simulink model "bus_as_currsource_charging_discharging_final_rearranged"  (R2023a)
settings: Solver=VariableStepAuto  StartTime=0.0  StopTime=10.0  RelTol=1e-3
libraries: spsParallelRLCBranchLib x72, spsCurrentMeasurementLib x27, spsVoltageMeasurementLib x27, spspowerguiLib x25, spsControlledVoltageSourceLib x24, spsVariableResistorLib x24, spsSeriesRLCBranchLib x6, spsMosfetLib x2, sdolib x1, spsControlledCurrentSourceLib x1, spsGroundLib x1
(part 1 of 4)
settings Model: Creator=Amith  LastModifiedBy=Amith

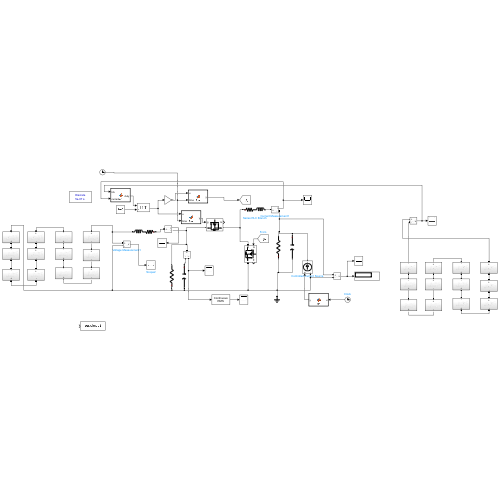
[thumbnail: Simulink's stored preview of the top-level diagram]
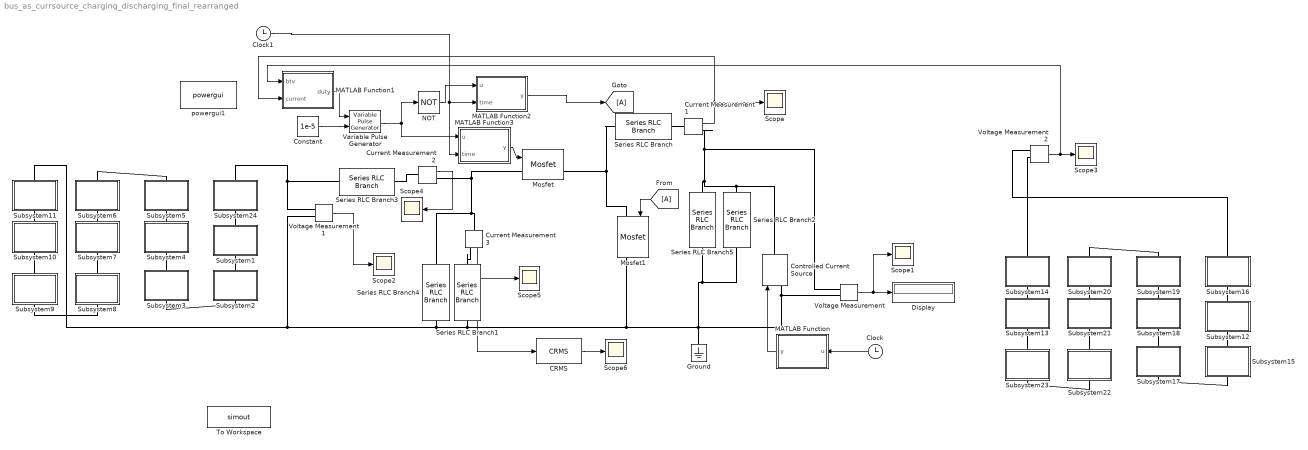
== system bus_as_currsource_charging_discharging_final_rearranged ==
  CRMS : sdolib/RMS Blocks/CRMS
  Clock : Clock
  Clock1 : Clock
  Constant : Constant  Value=1e-5
  Controlled Current Source : spsControlledCurrentSourceLib/Controlled Current Source  Initialize=on  Source_Type=AC  Amplitude=0  Phase=0  Frequency=0  Measurements=None
  Current Measurement1 : spsCurrentMeasurementLib/Current Measurement  PhasorSimulation=off  OutputType=Complex  PSBequivalent=0
  Current Measurement2 : spsCurrentMeasurementLib/Current Measurement  PhasorSimulation=off  OutputType=Complex  PSBequivalent=0
  Current Measurement3 : spsCurrentMeasurementLib/Current Measurement  PhasorSimulation=off  OutputType=Complex  PSBequivalent=0
  Display : Display
  From : From
  Goto : Goto
  Ground : spsGroundLib/Ground  LConnTagsString=a
  MATLAB Function : MATLAB Function  TreatAsAtomicUnit=on
  MATLAB Function1 : MATLAB Function  TreatAsAtomicUnit=on
  MATLAB Function2 : MATLAB Function  TreatAsAtomicUnit=on
  MATLAB Function3 : MATLAB Function  TreatAsAtomicUnit=on
  Mosfet : spsMosfetLib/Mosfet  Ron=0.1  Lon=0  Rd=0.01  Vfd=0  IC=0  Rs=1e5  Cs=inf  Measurements=on
  Mosfet1 : spsMosfetLib/Mosfet  Ron=0.1  Lon=0  Rd=0.01  Vfd=0  IC=0  Rs=1e5  Cs=inf  Measurements=on
  NOT : Logic  Operator=NOT  IconShape=distinctive  AllPortsSameDT=off  OutDataTypeStr=boolean
  Scope{,1..6} (7 alike) : Scope
  Series RLC Branch : spsSeriesRLCBranchLib/Series RLC Branch  LConnTagsString=__new0  RConnTagsString=__new0  BranchType=RL  Resistance=2.4e-3  Inductance=22e-6  SetiL0=off  InitialCurrent=0  Capacitance=1e-6  Setx0=off  InitialVoltage=0  Measurements=None
  Series RLC Branch1 : spsSeriesRLCBranchLib/Series RLC Branch  LConnTagsString=__new0  RConnTagsString=__new0  BranchType=C  Resistance=1  Inductance=1e-3  SetiL0=off  InitialCurrent=0  Capacitance=94e-6  Setx0=off  InitialVoltage=0  Measurements=None
  Series RLC Branch2 : spsSeriesRLCBranchLib/Series RLC Branch  LConnTagsString=__new0  RConnTagsString=__new0  BranchType=C  Resistance=1  Inductance=1e-3  SetiL0=off  InitialCurrent=0  Capacitance=188e-6  Setx0=off  InitialVoltage=0  Measurements=None
  Series RLC Branch3 : spsSeriesRLCBranchLib/Series RLC Branch  LConnTagsString=__new0  RConnTagsString=__new0  BranchType=RL  Resistance=2.4e-3  Inductance=22e-6  SetiL0=off  InitialCurrent=0  Capacitance=256.86e-6  Setx0=off  InitialVoltage=0  Measurements=None
  Series RLC Branch4 : spsSeriesRLCBranchLib/Series RLC Branch  LConnTagsString=__new0  RConnTagsString=__new0  BranchType=R  Resistance=10e3  Inductance=22e-6  SetiL0=off  InitialCurrent=0  Capacitance=256.86e-6  Setx0=off  InitialVoltage=0  Measurements=None
  Series RLC Branch5 : spsSeriesRLCBranchLib/Series RLC Branch  LConnTagsString=__new0  RConnTagsString=__new0  BranchType=R  Resistance=10e3  Inductance=22e-6  SetiL0=off  InitialCurrent=0  Capacitance=256.86e-6  Setx0=off  InitialVoltage=0  Measurements=None
  Subsystem1 : Subsystem
  Subsystem10 : Subsystem
  Subsystem11 : Subsystem
  Subsystem12 : Subsystem
  Subsystem13 : Subsystem
  Subsystem14 : Subsystem
  Subsystem15 : Subsystem
  Subsystem16 : Subsystem
  Subsystem17 : Subsystem
  Subsystem18 : Subsystem
  Subsystem19 : Subsystem
  Subsystem2 : Subsystem
  Subsystem20 : Subsystem
  Subsystem21 : Subsystem
  Subsystem22 : Subsystem
  Subsystem23 : Subsystem
  Subsystem24 : Subsystem
  Subsystem3 : Subsystem
  Subsystem4 : Subsystem
  Subsystem5 : Subsystem
  Subsystem6 : Subsystem
  Subsystem7 : Subsystem
  Subsystem8 : Subsystem
  Subsystem9 : Subsystem
  To Workspace : ToWorkspace  VariableName=simout  SaveFormat=Timeseries  SampleTime=-1
  Variable Pulse Generator : VariablePulseGenerator  SampleTime=0.1
  Voltage Measurement : spsVoltageMeasurementLib/Voltage Measurement  PhasorSimulation=off  OutputType=Complex  PSBequivalent=0
  Voltage Measurement1 : spsVoltageMeasurementLib/Voltage Measurement  PhasorSimulation=off  OutputType=Complex  PSBequivalent=0
  Voltage Measurement2 : spsVoltageMeasurementLib/Voltage Measurement  PhasorSimulation=off  OutputType=Complex  PSBequivalent=0
  powergui1 : spspowerguiLib/powergui  Priority=1  SimulationMode=Discrete  SampleTime=5e-7  frequency=60  Iterations=50  frequencyindice=0  Pbase=100e6  ErrMax=1e-4  UnitsV=kV  UnitsW=MW  buscounter=0  FunctionMessages=off  echomessages=off  EnableUseOfTLC=off  CurrentSourceSwitches=off  DisableSnubberDevices=off  DisableRonSwitches=off  DisableVfSwitches=off  DisplayEquations=off  AutomaticDiscreteSolvers=off  SolverType=Tustin/Backward Euler (TBE)  Interpol=off  ExternalGateDelay=off  methode=off  Ts=100  x0status=blocks  SPID=on  SwTol=0  HookPort=off  NonlinearTolerance=1e-4  nMaxIteration=100  ContinueOnMaxIteration=off  RestoreLinks=warning  ResistiveCurrentMeasurement=off  Frange=[0:2:500]  Ylog=off  Xlog=on  ShowGrid=off  save=off  variable=ZData  structure=0  ZoomFFT=off  StartTime=0.0  cycles=1  DisplayStyle=1  fundamental=60  FreqAxis=off  MaxFrequency=1000  frequencyindicesteady=1  RmsSteady=1  display=off
  wires:
  Voltage Measurement/1 -> Scope1/1, Display/1
  MATLAB Function1/1(duty) -> Variable Pulse Generator/1
  Clock/1 -> MATLAB Function/1(u)
  Current Measurement2/1 -> Scope4/1
  From/1 -> Mosfet1/1
  Constant/1 -> Variable Pulse Generator/2
  Current Measurement3/1 -> Scope5/1, CRMS/1
  CRMS/1 -> Scope6/1
  NOT/1 -> MATLAB Function2/1(u)
  Current Measurement1/1 -> Scope/1, MATLAB Function1/2(current)
  MATLAB Function2/1(y) -> Goto/1
  MATLAB Function/1(y) -> Controlled Current Source/1
  MATLAB Function3/1(y) -> Mosfet/1
  Clock1/1 -> MATLAB Function3/2(time), MATLAB Function2/2(time)
  Variable Pulse Generator/1 -> MATLAB Function3/1(u), NOT/1
  Voltage Measurement2/1 -> MATLAB Function1/1(btv), Scope3/1
  Voltage Measurement1/1 -> Scope2/1
  connections:
  Series RLC Branch2/RConn1 -- Voltage Measurement/LConn2 -- Controlled Current Source/LConn1 -- Ground/LConn1 -- Subsystem11/LConn1 -- Voltage Measurement1/LConn2 -- Series RLC Branch4/LConn1 -- Series RLC Branch1/RConn1 -- Mosfet1/RConn1 -- Series RLC Branch5/LConn1
  Current Measurement1/RConn1 -- Voltage Measurement/LConn1 -- Controlled Current Source/RConn1 -- Series RLC Branch2/LConn1 -- Series RLC Branch5/RConn1
  Series RLC Branch3/RConn1 -- Voltage Measurement1/LConn1 -- Subsystem24/RConn1
  Mosfet/RConn1 -- Mosfet1/LConn1 -- Series RLC Branch/LConn1
  Current Measurement3/LConn1 -- Series RLC Branch4/RConn1 -- Current Measurement2/RConn1 -- Mosfet/LConn1
  Subsystem15/LConn1 -- Subsystem17/RConn1
  Subsystem16/RConn1 -- Voltage Measurement2/LConn1
  Subsystem7/RConn1 -- Subsystem6/LConn1
  Subsystem8/LConn1 -- Subsystem9/RConn1
  Subsystem12/RConn1 -- Subsystem16/LConn1
  Subsystem22/LConn1 -- Subsystem23/RConn1
  Subsystem20/RConn1 -- Subsystem19/LConn1
  Subsystem8/RConn1 -- Subsystem7/LConn1
  Subsystem4/RConn1 -- Subsystem3/LConn1
  Subsystem2/RConn1 -- Subsystem1/LConn1
  Subsystem11/RConn1 -- Subsystem10/LConn1
  Subsystem13/RConn1 -- Subsystem23/LConn1
  Subsystem19/RConn1 -- Subsystem18/LConn1
  Subsystem14/RConn1 -- Subsystem13/LConn1
  Subsystem18/RConn1 -- Subsystem17/LConn1
  Current Measurement1/LConn1 -- Series RLC Branch/RConn1
  Subsystem5/RConn1 -- Subsystem4/LConn1
  Subsystem1/RConn1 -- Subsystem24/LConn1
  Subsystem10/RConn1 -- Subsystem9/LConn1
  Current Measurement2/LConn1 -- Series RLC Branch3/LConn1
  Subsystem15/RConn1 -- Subsystem12/LConn1
  Subsystem14/LConn1 -- Voltage Measurement2/LConn2
  Series RLC Branch1/LConn1 -- Current Measurement3/RConn1
  Subsystem22/RConn1 -- Subsystem21/LConn1
  Subsystem6/RConn1 -- Subsystem5/LConn1
  Subsystem3/RConn1 -- Subsystem2/LConn1
  Subsystem21/RConn1 -- Subsystem20/LConn1

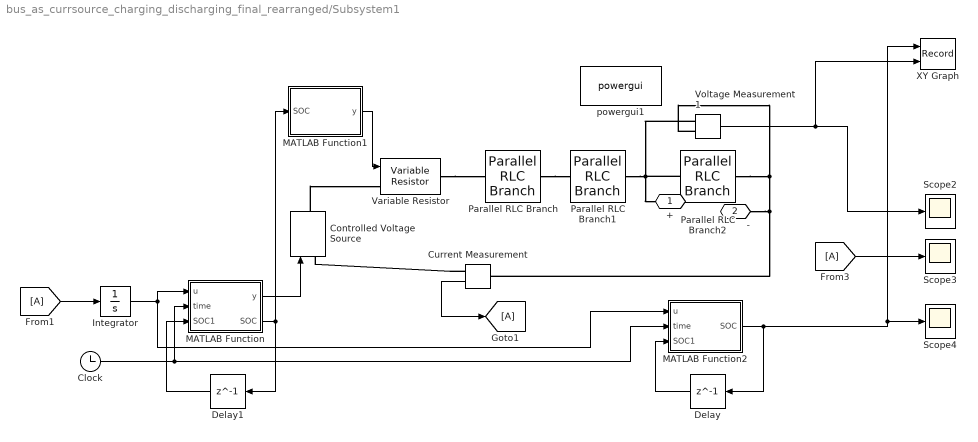
== system bus_as_currsource_charging_discharging_final_rearranged/Subsystem1 ==
  Clock : Clock
  Controlled Voltage Source : spsControlledVoltageSourceLib/Controlled Voltage Source  Initialize=on  Source_Type=DC  Amplitude=0  Phase=0  Frequency=0  Measurements=None
  Current Measurement : spsCurrentMeasurementLib/Current Measurement  PhasorSimulation=off  OutputType=Complex  PSBequivalent=0
  Delay : Delay  DelayLength=1  InitialCondition=0
  Delay1 : Delay  DelayLength=1  InitialCondition=0
  From1 : From
  From3 : From
  Goto1 : Goto
  Integrator : Integrator
  MATLAB Function : MATLAB Function  TreatAsAtomicUnit=on
  MATLAB Function1 : MATLAB Function  TreatAsAtomicUnit=on
  MATLAB Function2 : MATLAB Function  TreatAsAtomicUnit=on
  Parallel RLC Branch : spsParallelRLCBranchLib/Parallel RLC Branch  LConnTagsString=a  RConnTagsString=__new0  BranchType=RC  Resistance=15.5e-3  Inductance=1e-3  SetiL0=off  InitialCurrent=0  Capacitance=1028.7  Setx0=off  InitialVoltage=0  Measurements=None
  Parallel RLC Branch1 : spsParallelRLCBranchLib/Parallel RLC Branch  LConnTagsString=a  RConnTagsString=__new0  BranchType=RC  Resistance=18.3e-3  Inductance=1e-3  SetiL0=off  InitialCurrent=0  Capacitance=5756.6  Setx0=off  InitialVoltage=0  Measurements=None
  Parallel RLC Branch2 : spsParallelRLCBranchLib/Parallel RLC Branch  LConnTagsString=a  RConnTagsString=__new0  BranchType=R  Resistance=1e9  Inductance=1e-3  SetiL0=off  InitialCurrent=0  Capacitance=5756.6  Setx0=off  InitialVoltage=0  Measurements=None
  Scope2 : Scope
  Scope3 : Scope
  Scope4 : Scope
  Variable Resistor : spsVariableResistorLib/Variable Resistor  Rabsmin=1e-3
      settings: LibrarySourceBlock=sps_lib/Passives/Variable Resistor
  Voltage Measurement1 : spsVoltageMeasurementLib/Voltage Measurement  PhasorSimulation=off  OutputType=Complex  PSBequivalent=0
  XY Graph : Record  FileSettingsInternal="{\"entries\":[{\"content\":{\"excelSettings\":{\"content\":{},\"type\":\"Streamout.ExcelSettings\"}},\"type\":\"Streamout.FileSettingStorage\",\"uuid\":\"18842006-f205-45f0-aa2a-5042201a1171\"}],\"packageUris\":[\"http://schema.mathworks.com/mf0/streamout_blocks/R2020a\"],\"version\":\"1.0\"}"  Layout=[1 1]  SignalsInternal="{\"entries\":[{\"content\":{\"signals\":[{\"content\":{\"blockPath\":[\"untitled/Subsystem1/XY Graph\"],\"dimensions\":[1],\"domain\":\"untitled/Subsystem1/XY Graph\",\"lineColor\":\"#a2142f\",\"port\":1,\"signalID\":718,\"signalName\":\"MATLAB Function2\"},\"type\":\"RecordBlkView.Signal\",\"uuid\":\"8255158c-12c1-48e7-a974-9ade2a17e088\"},{\"content\":{\"blockPath\":[\"untitled/Subsystem1/XY Graph\"],\"dimensions\":[1],\"domain\":\"untitled/Subsystem1/XY Graph\",\"lineColor\":\"#139fff\",\"port\":2,\"signalID\":721,\"signalName\":\"Voltage Measurement1\"},\"type\":\"RecordBlkView.Signal\",\"uuid\":\"5dae4a47-f7fb-4179-ba61-09f1c7b2ee25\"}]},\"type\":\"RecordBlkView.InputSignals\",\"uuid\":\"df1e2d31-8fbb-4e56-9ead-2e4de2629ece\"}],\"packageUris\":[\"http://schema.mathworks.com/mf0/streamout_blocks/R2020a\"],\"version\":\"1.0\"}"  VisualizationBindings="{\"xyplotplugin\":{\"info\":[{\"series\":[],\"subplotID\":1}]}}"  CompatibilityTag=XY
  powergui1 : spspowerguiLib/powergui  Priority=1  SimulationMode=Discrete  SampleTime=2e-7  frequency=60  Iterations=50  frequencyindice=0  Pbase=100e6  ErrMax=1e-4  UnitsV=kV  UnitsW=MW  buscounter=0  FunctionMessages=off  echomessages=off  EnableUseOfTLC=off  CurrentSourceSwitches=off  DisableSnubberDevices=off  DisableRonSwitches=off  DisableVfSwitches=off  DisplayEquations=off  AutomaticDiscreteSolvers=off  SolverType=Tustin/Backward Euler (TBE)  Interpol=off  ExternalGateDelay=off  methode=off  Ts=100  x0status=blocks  SPID=on  SwTol=0  HookPort=off  NonlinearTolerance=1e-4  nMaxIteration=100  ContinueOnMaxIteration=off  RestoreLinks=warning  ResistiveCurrentMeasurement=off  Frange=[0:2:500]  Ylog=off  Xlog=on  ShowGrid=off  save=off  variable=ZData  structure=0  ZoomFFT=off  StartTime=0.0  cycles=1  DisplayStyle=1  fundamental=60  FreqAxis=off  MaxFrequency=1000  frequencyindicesteady=1  RmsSteady=1  display=off
  + : PMIOPort  Side=Right
  - : PMIOPort  Port=2  Side=Left
  wires:
  Current Measurement/1 -> Goto1/1
  From3/1 -> Scope3/1
  Voltage Measurement1/1 -> XY Graph/2, Scope2/1
  MATLAB Function2/1(SOC) -> Delay/1, XY Graph/1, Scope4/1
  From1/1 -> Integrator/1
  MATLAB Function/1(y) -> Controlled Voltage Source/1
  MATLAB Function1/1(y) -> Variable Resistor/1
  Integrator/1 -> MATLAB Function2/1(u), MATLAB Function/1(u)
  Clock/1 -> MATLAB Function2/2(time), MATLAB Function/2(time)
  MATLAB Function/2(SOC) -> Delay1/1, MATLAB Function1/1(SOC)
  Delay/1 -> MATLAB Function2/3(SOC1)
  Delay1/1 -> MATLAB Function/3(SOC1)
  connections:
  Variable Resistor/RConn1 -- Parallel RLC Branch/LConn1
  Parallel RLC Branch1/RConn1 -- Parallel RLC Branch2/LConn1 -- +/RConn1 -- Voltage Measurement1/LConn1
  Voltage Measurement1/LConn2 -- Parallel RLC Branch2/RConn1 -- -/RConn1 -- Current Measurement/LConn1
  Controlled Voltage Source/RConn1 -- Variable Resistor/LConn1
  Current Measurement/RConn1 -- Controlled Voltage Source/LConn1
  Parallel RLC Branch/RConn1 -- Parallel RLC Branch1/LConn1

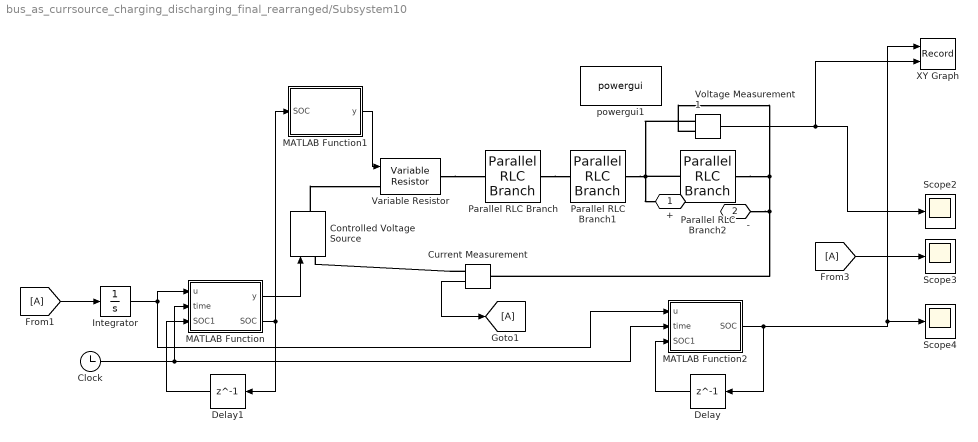
== system bus_as_currsource_charging_discharging_final_rearranged/Subsystem10 ==
  Clock : Clock
  Controlled Voltage Source : spsControlledVoltageSourceLib/Controlled Voltage Source  Initialize=on  Source_Type=DC  Amplitude=0  Phase=0  Frequency=0  Measurements=None
  Current Measurement : spsCurrentMeasurementLib/Current Measurement  PhasorSimulation=off  OutputType=Complex  PSBequivalent=0
  Delay : Delay  DelayLength=1  InitialCondition=0
  Delay1 : Delay  DelayLength=1  InitialCondition=0
  From1 : From
  From3 : From
  Goto1 : Goto
  Integrator : Integrator
  MATLAB Function : MATLAB Function  TreatAsAtomicUnit=on
  MATLAB Function1 : MATLAB Function  TreatAsAtomicUnit=on
  MATLAB Function2 : MATLAB Function  TreatAsAtomicUnit=on
  Parallel RLC Branch : spsParallelRLCBranchLib/Parallel RLC Branch  LConnTagsString=a  RConnTagsString=__new0  BranchType=RC  Resistance=15.5e-3  Inductance=1e-3  SetiL0=off  InitialCurrent=0  Capacitance=1028.7  Setx0=off  InitialVoltage=0  Measurements=None
  Parallel RLC Branch1 : spsParallelRLCBranchLib/Parallel RLC Branch  LConnTagsString=a  RConnTagsString=__new0  BranchType=RC  Resistance=18.3e-3  Inductance=1e-3  SetiL0=off  InitialCurrent=0  Capacitance=5756.6  Setx0=off  InitialVoltage=0  Measurements=None
  Parallel RLC Branch2 : spsParallelRLCBranchLib/Parallel RLC Branch  LConnTagsString=a  RConnTagsString=__new0  BranchType=R  Resistance=1e9  Inductance=1e-3  SetiL0=off  InitialCurrent=0  Capacitance=5756.6  Setx0=off  InitialVoltage=0  Measurements=None
  Scope2 : Scope
  Scope3 : Scope
  Scope4 : Scope
  Variable Resistor : spsVariableResistorLib/Variable Resistor  Rabsmin=1e-3
      settings: LibrarySourceBlock=sps_lib/Passives/Variable Resistor
  Voltage Measurement1 : spsVoltageMeasurementLib/Voltage Measurement  PhasorSimulation=off  OutputType=Complex  PSBequivalent=0
  XY Graph : Record  FileSettingsInternal="{\"entries\":[{\"content\":{\"excelSettings\":{\"content\":{},\"type\":\"Streamout.ExcelSettings\"}},\"type\":\"Streamout.FileSettingStorage\",\"uuid\":\"22b4d28b-aa9d-4c7b-bafe-c9a2b3ab8659\"}],\"packageUris\":[\"http://schema.mathworks.com/mf0/streamout_blocks/R2020a\"],\"version\":\"1.0\"}"  Layout=[1 1]  SignalsInternal="{\"entries\":[{\"content\":{\"signals\":[{\"content\":{\"blockPath\":[\"untitled/Subsystem10/XY Graph\"],\"dimensions\":[1],\"domain\":\"untitled/Subsystem10/XY Graph\",\"lineColor\":\"#ff6929\",\"port\":1,\"signalID\":726,\"signalName\":\"MATLAB Function2\"},\"type\":\"RecordBlkView.Signal\",\"uuid\":\"416f6dc6-347a-4c18-b72a-d27e661ecc55\"},{\"content\":{\"blockPath\":[\"untitled/Subsystem10/XY Graph\"],\"dimensions\":[1],\"domain\":\"untitled/Subsystem10/XY Graph\",\"lineColor\":\"#b746ff\",\"port\":2,\"signalID\":729,\"signalName\":\"Voltage Measurement1\"},\"type\":\"RecordBlkView.Signal\",\"uuid\":\"51357560-055d-4b10-b7e9-279a1a15faeb\"}]},\"type\":\"RecordBlkView.InputSignals\",\"uuid\":\"f10ebc27-9336-481b-9fb2-eb231a30c92e\"}],\"packageUris\":[\"http://schema.mathworks.com/mf0/streamout_blocks/R2020a\"],\"version\":\"1.0\"}"  VisualizationBindings="{\"xyplotplugin\":{\"info\":[{\"series\":[],\"subplotID\":1}]}}"  CompatibilityTag=XY
  powergui1 : spspowerguiLib/powergui  Priority=1  SimulationMode=Discrete  SampleTime=2e-7  frequency=60  Iterations=50  frequencyindice=0  Pbase=100e6  ErrMax=1e-4  UnitsV=kV  UnitsW=MW  buscounter=0  FunctionMessages=off  echomessages=off  EnableUseOfTLC=off  CurrentSourceSwitches=off  DisableSnubberDevices=off  DisableRonSwitches=off  DisableVfSwitches=off  DisplayEquations=off  AutomaticDiscreteSolvers=off  SolverType=Tustin/Backward Euler (TBE)  Interpol=off  ExternalGateDelay=off  methode=off  Ts=100  x0status=blocks  SPID=on  SwTol=0  HookPort=off  NonlinearTolerance=1e-4  nMaxIteration=100  ContinueOnMaxIteration=off  RestoreLinks=warning  ResistiveCurrentMeasurement=off  Frange=[0:2:500]  Ylog=off  Xlog=on  ShowGrid=off  save=off  variable=ZData  structure=0  ZoomFFT=off  StartTime=0.0  cycles=1  DisplayStyle=1  fundamental=60  FreqAxis=off  MaxFrequency=1000  frequencyindicesteady=1  RmsSteady=1  display=off
  + : PMIOPort  Side=Right
  - : PMIOPort  Port=2  Side=Left
  wires:
  Current Measurement/1 -> Goto1/1
  From3/1 -> Scope3/1
  Voltage Measurement1/1 -> XY Graph/2, Scope2/1
  MATLAB Function2/1(SOC) -> Delay/1, XY Graph/1, Scope4/1
  From1/1 -> Integrator/1
  MATLAB Function/1(y) -> Controlled Voltage Source/1
  MATLAB Function1/1(y) -> Variable Resistor/1
  Integrator/1 -> MATLAB Function2/1(u), MATLAB Function/1(u)
  Clock/1 -> MATLAB Function2/2(time), MATLAB Function/2(time)
  MATLAB Function/2(SOC) -> Delay1/1, MATLAB Function1/1(SOC)
  Delay/1 -> MATLAB Function2/3(SOC1)
  Delay1/1 -> MATLAB Function/3(SOC1)
  connections:
  Variable Resistor/RConn1 -- Parallel RLC Branch/LConn1
  Parallel RLC Branch1/RConn1 -- Parallel RLC Branch2/LConn1 -- +/RConn1 -- Voltage Measurement1/LConn1
  Voltage Measurement1/LConn2 -- Parallel RLC Branch2/RConn1 -- -/RConn1 -- Current Measurement/LConn1
  Controlled Voltage Source/RConn1 -- Variable Resistor/LConn1
  Current Measurement/RConn1 -- Controlled Voltage Source/LConn1
  Parallel RLC Branch/RConn1 -- Parallel RLC Branch1/LConn1

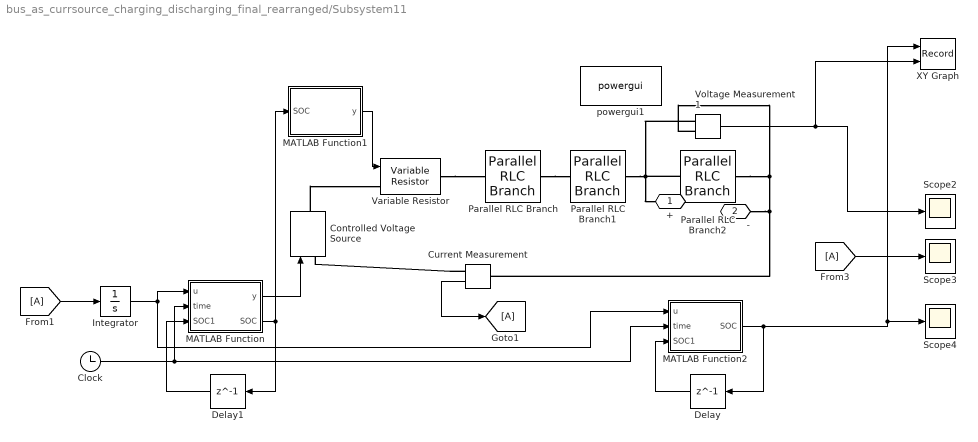
== system bus_as_currsource_charging_discharging_final_rearranged/Subsystem11 ==
  Clock : Clock
  Controlled Voltage Source : spsControlledVoltageSourceLib/Controlled Voltage Source  Initialize=on  Source_Type=DC  Amplitude=0  Phase=0  Frequency=0  Measurements=None
  Current Measurement : spsCurrentMeasurementLib/Current Measurement  PhasorSimulation=off  OutputType=Complex  PSBequivalent=0
  Delay : Delay  DelayLength=1  InitialCondition=0
  Delay1 : Delay  DelayLength=1  InitialCondition=0
  From1 : From
  From3 : From
  Goto1 : Goto
  Integrator : Integrator
  MATLAB Function : MATLAB Function  TreatAsAtomicUnit=on
  MATLAB Function1 : MATLAB Function  TreatAsAtomicUnit=on
  MATLAB Function2 : MATLAB Function  TreatAsAtomicUnit=on
  Parallel RLC Branch : spsParallelRLCBranchLib/Parallel RLC Branch  LConnTagsString=a  RConnTagsString=__new0  BranchType=RC  Resistance=15.5e-3  Inductance=1e-3  SetiL0=off  InitialCurrent=0  Capacitance=1028.7  Setx0=off  InitialVoltage=0  Measurements=None
  Parallel RLC Branch1 : spsParallelRLCBranchLib/Parallel RLC Branch  LConnTagsString=a  RConnTagsString=__new0  BranchType=RC  Resistance=18.3e-3  Inductance=1e-3  SetiL0=off  InitialCurrent=0  Capacitance=5756.6  Setx0=off  InitialVoltage=0  Measurements=None
  Parallel RLC Branch2 : spsParallelRLCBranchLib/Parallel RLC Branch  LConnTagsString=a  RConnTagsString=__new0  BranchType=R  Resistance=1e9  Inductance=1e-3  SetiL0=off  InitialCurrent=0  Capacitance=5756.6  Setx0=off  InitialVoltage=0  Measurements=None
  Scope2 : Scope
  Scope3 : Scope
  Scope4 : Scope
  Variable Resistor : spsVariableResistorLib/Variable Resistor  Rabsmin=1e-3
      settings: LibrarySourceBlock=sps_lib/Passives/Variable Resistor
  Voltage Measurement1 : spsVoltageMeasurementLib/Voltage Measurement  PhasorSimulation=off  OutputType=Complex  PSBequivalent=0
  XY Graph : Record  FileSettingsInternal="{\"entries\":[{\"content\":{\"excelSettings\":{\"content\":{},\"type\":\"Streamout.ExcelSettings\"}},\"type\":\"Streamout.FileSettingStorage\",\"uuid\":\"1c848b0b-adcf-4d1f-b91d-bbb3ed9b825d\"}],\"packageUris\":[\"http://schema.mathworks.com/mf0/streamout_blocks/R2020a\"],\"version\":\"1.0\"}"  Layout=[1 1]  SignalsInternal="{\"entries\":[{\"content\":{\"signals\":[{\"content\":{\"blockPath\":[\"untitled/Subsystem11/XY Graph\"],\"dimensions\":[1],\"domain\":\"untitled/Subsystem11/XY Graph\",\"lineColor\":\"#64d413\",\"port\":1,\"signalID\":734,\"signalName\":\"MATLAB Function2\"},\"type\":\"RecordBlkView.Signal\",\"uuid\":\"47c9a702-d54e-4048-aa36-620fba24fcff\"},{\"content\":{\"blockPath\":[\"untitled/Subsystem11/XY Graph\"],\"dimensions\":[1],\"domain\":\"untitled/Subsystem11/XY Graph\",\"lineColor\":\"#ff13a6\",\"port\":2,\"signalID\":737,\"signalName\":\"Voltage Measurement1\"},\"type\":\"RecordBlkView.Signal\",\"uuid\":\"f7e45941-7ce1-4a94-86f8-fd3d3864fbc4\"}]},\"type\":\"RecordBlkView.InputSignals\",\"uuid\":\"d32c99c7-d674-4a48-9e7c-b1b0ccc14c0d\"}],\"packageUris\":[\"http://schema.mathworks.com/mf0/streamout_blocks/R2020a\"],\"version\":\"1.0\"}"  VisualizationBindings="{\"xyplotplugin\":{\"info\":[{\"series\":[],\"subplotID\":1}]}}"  CompatibilityTag=XY
  powergui1 : spspowerguiLib/powergui  Priority=1  SimulationMode=Discrete  SampleTime=2e-7  frequency=60  Iterations=50  frequencyindice=0  Pbase=100e6  ErrMax=1e-4  UnitsV=kV  UnitsW=MW  buscounter=0  FunctionMessages=off  echomessages=off  EnableUseOfTLC=off  CurrentSourceSwitches=off  DisableSnubberDevices=off  DisableRonSwitches=off  DisableVfSwitches=off  DisplayEquations=off  AutomaticDiscreteSolvers=off  SolverType=Tustin/Backward Euler (TBE)  Interpol=off  ExternalGateDelay=off  methode=off  Ts=100  x0status=blocks  SPID=on  SwTol=0  HookPort=off  NonlinearTolerance=1e-4  nMaxIteration=100  ContinueOnMaxIteration=off  RestoreLinks=warning  ResistiveCurrentMeasurement=off  Frange=[0:2:500]  Ylog=off  Xlog=on  ShowGrid=off  save=off  variable=ZData  structure=0  ZoomFFT=off  StartTime=0.0  cycles=1  DisplayStyle=1  fundamental=60  FreqAxis=off  MaxFrequency=1000  frequencyindicesteady=1  RmsSteady=1  display=off
  + : PMIOPort  Side=Right
  - : PMIOPort  Port=2  Side=Left
  wires:
  Current Measurement/1 -> Goto1/1
  From3/1 -> Scope3/1
  Voltage Measurement1/1 -> XY Graph/2, Scope2/1
  MATLAB Function2/1(SOC) -> Delay/1, XY Graph/1, Scope4/1
  From1/1 -> Integrator/1
  MATLAB Function/1(y) -> Controlled Voltage Source/1
  MATLAB Function1/1(y) -> Variable Resistor/1
  Integrator/1 -> MATLAB Function2/1(u), MATLAB Function/1(u)
  Clock/1 -> MATLAB Function2/2(time), MATLAB Function/2(time)
  MATLAB Function/2(SOC) -> Delay1/1, MATLAB Function1/1(SOC)
  Delay/1 -> MATLAB Function2/3(SOC1)
  Delay1/1 -> MATLAB Function/3(SOC1)
  connections:
  Variable Resistor/RConn1 -- Parallel RLC Branch/LConn1
  Parallel RLC Branch1/RConn1 -- Parallel RLC Branch2/LConn1 -- +/RConn1 -- Voltage Measurement1/LConn1
  Voltage Measurement1/LConn2 -- Parallel RLC Branch2/RConn1 -- -/RConn1 -- Current Measurement/LConn1
  Controlled Voltage Source/RConn1 -- Variable Resistor/LConn1
  Current Measurement/RConn1 -- Controlled Voltage Source/LConn1
  Parallel RLC Branch/RConn1 -- Parallel RLC Branch1/LConn1

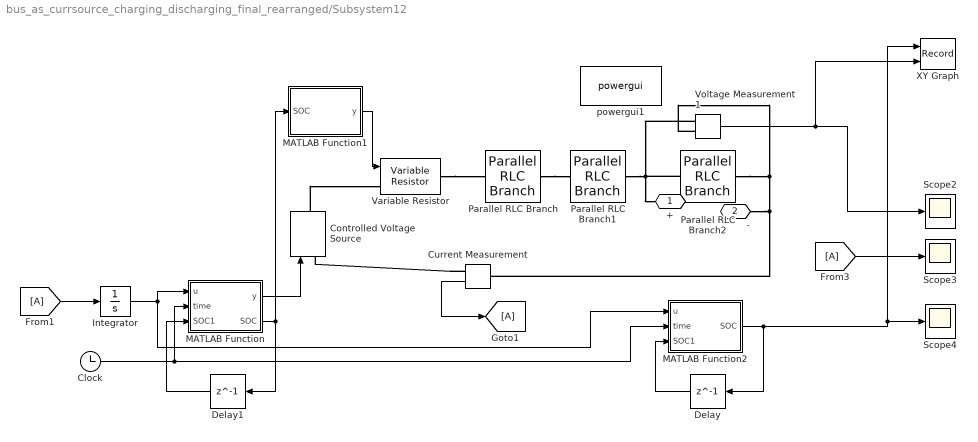
== system bus_as_currsource_charging_discharging_final_rearranged/Subsystem12 ==
  Clock : Clock
  Controlled Voltage Source : spsControlledVoltageSourceLib/Controlled Voltage Source  Initialize=on  Source_Type=DC  Amplitude=0  Phase=0  Frequency=0  Measurements=None
  Current Measurement : spsCurrentMeasurementLib/Current Measurement  PhasorSimulation=off  OutputType=Complex  PSBequivalent=0
  Delay : Delay  DelayLength=1  InitialCondition=0
  Delay1 : Delay  DelayLength=1  InitialCondition=0
  From1 : From
  From3 : From
  Goto1 : Goto
  Integrator : Integrator
  MATLAB Function : MATLAB Function  TreatAsAtomicUnit=on
  MATLAB Function1 : MATLAB Function  TreatAsAtomicUnit=on
  MATLAB Function2 : MATLAB Function  TreatAsAtomicUnit=on
  Parallel RLC Branch : spsParallelRLCBranchLib/Parallel RLC Branch  LConnTagsString=a  RConnTagsString=__new0  BranchType=RC  Resistance=15.5e-3  Inductance=1e-3  SetiL0=off  InitialCurrent=0  Capacitance=1028.7  Setx0=off  InitialVoltage=0  Measurements=None
  Parallel RLC Branch1 : spsParallelRLCBranchLib/Parallel RLC Branch  LConnTagsString=a  RConnTagsString=__new0  BranchType=RC  Resistance=18.3e-3  Inductance=1e-3  SetiL0=off  InitialCurrent=0  Capacitance=5756.6  Setx0=off  InitialVoltage=0  Measurements=None
  Parallel RLC Branch2 : spsParallelRLCBranchLib/Parallel RLC Branch  LConnTagsString=a  RConnTagsString=__new0  BranchType=R  Resistance=1e9  Inductance=1e-3  SetiL0=off  InitialCurrent=0  Capacitance=5756.6  Setx0=off  InitialVoltage=0  Measurements=None
  Scope2 : Scope
  Scope3 : Scope
  Scope4 : Scope
  Variable Resistor : spsVariableResistorLib/Variable Resistor  Rabsmin=1e-3
      settings: LibrarySourceBlock=sps_lib/Passives/Variable Resistor
  Voltage Measurement1 : spsVoltageMeasurementLib/Voltage Measurement  PhasorSimulation=off  OutputType=Complex  PSBequivalent=0
  XY Graph : Record  FileSettingsInternal="{\"entries\":[{\"content\":{\"excelSettings\":{\"content\":{},\"type\":\"Streamout.ExcelSettings\"}},\"type\":\"Streamout.FileSettingStorage\",\"uuid\":\"0f2e6bc2-adc7-4f2f-b180-28a43c082b9a\"}],\"packageUris\":[\"http://schema.mathworks.com/mf0/streamout_blocks/R2020a\"],\"version\":\"1.0\"}"  Layout=[1 1]  SignalsInternal="{\"entries\":[{\"content\":{\"signals\":[{\"content\":{\"blockPath\":[\"untitled/Subsystem12/XY Graph\"],\"dimensions\":[1],\"domain\":\"untitled/Subsystem12/XY Graph\",\"lineColor\":\"#fe330a\",\"port\":1,\"signalID\":742,\"signalName\":\"MATLAB Function2\"},\"type\":\"RecordBlkView.Signal\",\"uuid\":\"ea5ffbeb-f673-49b5-8228-f57bc36c2a28\"},{\"content\":{\"blockPath\":[\"untitled/Subsystem12/XY Graph\"],\"dimensions\":[1],\"domain\":\"untitled/Subsystem12/XY Graph\",\"lineColor\":\"#22b573\",\"port\":2,\"signalID\":745,\"signalName\":\"Voltage Measurement1\"},\"type\":\"RecordBlkView.Signal\",\"uuid\":\"e027727c-edef-4d69-b6da-103e96f1fdd0\"}]},\"type\":\"RecordBlkView.InputSignals\",\"uuid\":\"816a9515-beeb-4015-a901-a01888038e5f\"}],\"packageUris\":[\"http://schema.mathworks.com/mf0/streamout_blocks/R2020a\"],\"version\":\"1.0\"}"  VisualizationBindings="{\"xyplotplugin\":{\"info\":[{\"series\":[],\"subplotID\":1}]}}"  CompatibilityTag=XY
  powergui1 : spspowerguiLib/powergui  Priority=1  SimulationMode=Discrete  SampleTime=2e-7  frequency=60  Iterations=50  frequencyindice=0  Pbase=100e6  ErrMax=1e-4  UnitsV=kV  UnitsW=MW  buscounter=0  FunctionMessages=off  echomessages=off  EnableUseOfTLC=off  CurrentSourceSwitches=off  DisableSnubberDevices=off  DisableRonSwitches=off  DisableVfSwitches=off  DisplayEquations=off  AutomaticDiscreteSolvers=off  SolverType=Tustin/Backward Euler (TBE)  Interpol=off  ExternalGateDelay=off  methode=off  Ts=100  x0status=blocks  SPID=on  SwTol=0  HookPort=off  NonlinearTolerance=1e-4  nMaxIteration=100  ContinueOnMaxIteration=off  RestoreLinks=warning  ResistiveCurrentMeasurement=off  Frange=[0:2:500]  Ylog=off  Xlog=on  ShowGrid=off  save=off  variable=ZData  structure=0  ZoomFFT=off  StartTime=0.0  cycles=1  DisplayStyle=1  fundamental=60  FreqAxis=off  MaxFrequency=1000  frequencyindicesteady=1  RmsSteady=1  display=off
  + : PMIOPort  Side=Right
  - : PMIOPort  Port=2  Side=Left
  wires:
  Current Measurement/1 -> Goto1/1
  From3/1 -> Scope3/1
  Voltage Measurement1/1 -> XY Graph/2, Scope2/1
  MATLAB Function2/1(SOC) -> Delay/1, XY Graph/1, Scope4/1
  From1/1 -> Integrator/1
  MATLAB Function/1(y) -> Controlled Voltage Source/1
  MATLAB Function1/1(y) -> Variable Resistor/1
  Integrator/1 -> MATLAB Function2/1(u), MATLAB Function/1(u)
  Clock/1 -> MATLAB Function2/2(time), MATLAB Function/2(time)
  MATLAB Function/2(SOC) -> Delay1/1, MATLAB Function1/1(SOC)
  Delay/1 -> MATLAB Function2/3(SOC1)
  Delay1/1 -> MATLAB Function/3(SOC1)
  connections:
  Variable Resistor/RConn1 -- Parallel RLC Branch/LConn1
  Parallel RLC Branch1/RConn1 -- Parallel RLC Branch2/LConn1 -- +/RConn1 -- Voltage Measurement1/LConn1
  Voltage Measurement1/LConn2 -- Parallel RLC Branch2/RConn1 -- -/RConn1 -- Current Measurement/LConn1
  Controlled Voltage Source/RConn1 -- Variable Resistor/LConn1
  Current Measurement/RConn1 -- Controlled Voltage Source/LConn1
  Parallel RLC Branch/RConn1 -- Parallel RLC Branch1/LConn1

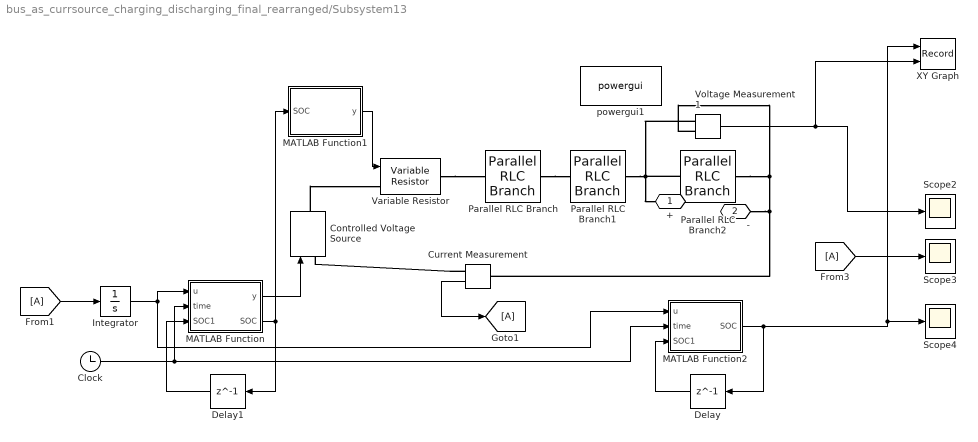
== system bus_as_currsource_charging_discharging_final_rearranged/Subsystem13 ==
  Clock : Clock
  Controlled Voltage Source : spsControlledVoltageSourceLib/Controlled Voltage Source  Initialize=on  Source_Type=DC  Amplitude=0  Phase=0  Frequency=0  Measurements=None
  Current Measurement : spsCurrentMeasurementLib/Current Measurement  PhasorSimulation=off  OutputType=Complex  PSBequivalent=0
  Delay : Delay  DelayLength=1  InitialCondition=0
  Delay1 : Delay  DelayLength=1  InitialCondition=0
  From1 : From
  From3 : From
  Goto1 : Goto
  Integrator : Integrator
  MATLAB Function : MATLAB Function  TreatAsAtomicUnit=on
  MATLAB Function1 : MATLAB Function  TreatAsAtomicUnit=on
  MATLAB Function2 : MATLAB Function  TreatAsAtomicUnit=on
  Parallel RLC Branch : spsParallelRLCBranchLib/Parallel RLC Branch  LConnTagsString=a  RConnTagsString=__new0  BranchType=RC  Resistance=15.5e-3  Inductance=1e-3  SetiL0=off  InitialCurrent=0  Capacitance=1028.7  Setx0=off  InitialVoltage=0  Measurements=None
  Parallel RLC Branch1 : spsParallelRLCBranchLib/Parallel RLC Branch  LConnTagsString=a  RConnTagsString=__new0  BranchType=RC  Resistance=18.3e-3  Inductance=1e-3  SetiL0=off  InitialCurrent=0  Capacitance=5756.6  Setx0=off  InitialVoltage=0  Measurements=None
  Parallel RLC Branch2 : spsParallelRLCBranchLib/Parallel RLC Branch  LConnTagsString=a  RConnTagsString=__new0  BranchType=R  Resistance=1e9  Inductance=1e-3  SetiL0=off  InitialCurrent=0  Capacitance=5756.6  Setx0=off  InitialVoltage=0  Measurements=None
  Scope2 : Scope
  Scope3 : Scope
  Scope4 : Scope
  Variable Resistor : spsVariableResistorLib/Variable Resistor  Rabsmin=1e-3
      settings: LibrarySourceBlock=sps_lib/Passives/Variable Resistor
  Voltage Measurement1 : spsVoltageMeasurementLib/Voltage Measurement  PhasorSimulation=off  OutputType=Complex  PSBequivalent=0
  XY Graph : Record  FileSettingsInternal="{\"entries\":[{\"content\":{\"excelSettings\":{\"content\":{},\"type\":\"Streamout.ExcelSettings\"}},\"type\":\"Streamout.FileSettingStorage\",\"uuid\":\"46f2ea04-5cee-4a3f-bbd1-60b3e0321189\"}],\"packageUris\":[\"http://schema.mathworks.com/mf0/streamout_blocks/R2020a\"],\"version\":\"1.0\"}"  Layout=[1 1]  SignalsInternal="{\"entries\":[{\"content\":{\"signals\":[{\"content\":{\"blockPath\":[\"untitled/Subsystem13/XY Graph\"],\"dimensions\":[1],\"domain\":\"untitled/Subsystem13/XY Graph\",\"lineColor\":\"#0072bd\",\"port\":1,\"signalID\":750,\"signalName\":\"MATLAB Function2\"},\"type\":\"RecordBlkView.Signal\",\"uuid\":\"17a12a08-f5f2-4398-835d-df73d8301e60\"},{\"content\":{\"blockPath\":[\"untitled/Subsystem13/XY Graph\"],\"dimensions\":[1],\"domain\":\"untitled/Subsystem13/XY Graph\",\"lineColor\":\"#d95319\",\"port\":2,\"signalID\":753,\"signalName\":\"Voltage Measurement1\"},\"type\":\"RecordBlkView.Signal\",\"uuid\":\"64892386-6769-470e-a7d8-214f68453155\"}]},\"type\":\"RecordBlkView.InputSignals\",\"uuid\":\"950e3db8-19c7-46df-8e03-320c742ac139\"}],\"packageUris\":[\"http://schema.mathworks.com/mf0/streamout_blocks/R2020a\"],\"version\":\"1.0\"}"  VisualizationBindings="{\"xyplotplugin\":{\"info\":[{\"series\":[],\"subplotID\":1}]}}"  CompatibilityTag=XY
  powergui1 : spspowerguiLib/powergui  Priority=1  SimulationMode=Discrete  SampleTime=2e-7  frequency=60  Iterations=50  frequencyindice=0  Pbase=100e6  ErrMax=1e-4  UnitsV=kV  UnitsW=MW  buscounter=0  FunctionMessages=off  echomessages=off  EnableUseOfTLC=off  CurrentSourceSwitches=off  DisableSnubberDevices=off  DisableRonSwitches=off  DisableVfSwitches=off  DisplayEquations=off  AutomaticDiscreteSolvers=off  SolverType=Tustin/Backward Euler (TBE)  Interpol=off  ExternalGateDelay=off  methode=off  Ts=100  x0status=blocks  SPID=on  SwTol=0  HookPort=off  NonlinearTolerance=1e-4  nMaxIteration=100  ContinueOnMaxIteration=off  RestoreLinks=warning  ResistiveCurrentMeasurement=off  Frange=[0:2:500]  Ylog=off  Xlog=on  ShowGrid=off  save=off  variable=ZData  structure=0  ZoomFFT=off  StartTime=0.0  cycles=1  DisplayStyle=1  fundamental=60  FreqAxis=off  MaxFrequency=1000  frequencyindicesteady=1  RmsSteady=1  display=off
  + : PMIOPort  Side=Right
  - : PMIOPort  Port=2  Side=Left
  wires:
  Current Measurement/1 -> Goto1/1
  From3/1 -> Scope3/1
  Voltage Measurement1/1 -> XY Graph/2, Scope2/1
  MATLAB Function2/1(SOC) -> Delay/1, XY Graph/1, Scope4/1
  From1/1 -> Integrator/1
  MATLAB Function/1(y) -> Controlled Voltage Source/1
  MATLAB Function1/1(y) -> Variable Resistor/1
  Integrator/1 -> MATLAB Function2/1(u), MATLAB Function/1(u)
  Clock/1 -> MATLAB Function2/2(time), MATLAB Function/2(time)
  MATLAB Function/2(SOC) -> Delay1/1, MATLAB Function1/1(SOC)
  Delay/1 -> MATLAB Function2/3(SOC1)
  Delay1/1 -> MATLAB Function/3(SOC1)
  connections:
  Variable Resistor/RConn1 -- Parallel RLC Branch/LConn1
  Parallel RLC Branch1/RConn1 -- Parallel RLC Branch2/LConn1 -- +/RConn1 -- Voltage Measurement1/LConn1
  Voltage Measurement1/LConn2 -- Parallel RLC Branch2/RConn1 -- -/RConn1 -- Current Measurement/LConn1
  Controlled Voltage Source/RConn1 -- Variable Resistor/LConn1
  Current Measurement/RConn1 -- Controlled Voltage Source/LConn1
  Parallel RLC Branch/RConn1 -- Parallel RLC Branch1/LConn1

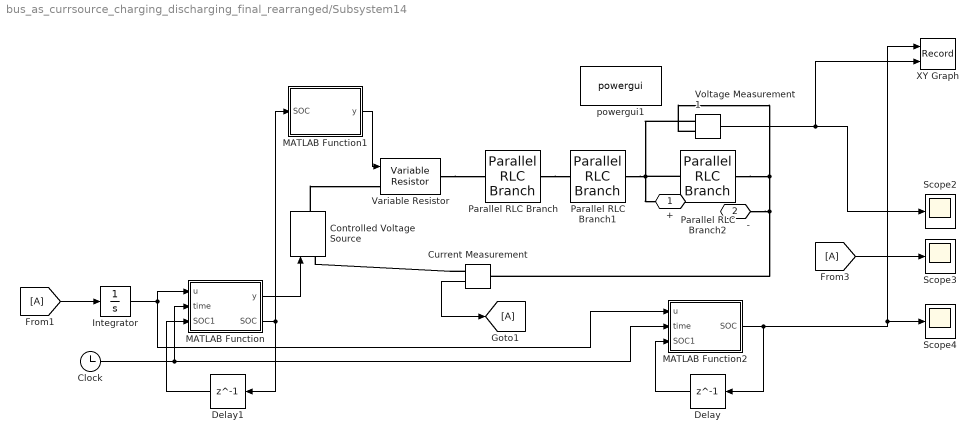
== system bus_as_currsource_charging_discharging_final_rearranged/Subsystem14 ==
  Clock : Clock
  Controlled Voltage Source : spsControlledVoltageSourceLib/Controlled Voltage Source  Initialize=on  Source_Type=DC  Amplitude=0  Phase=0  Frequency=0  Measurements=None
  Current Measurement : spsCurrentMeasurementLib/Current Measurement  PhasorSimulation=off  OutputType=Complex  PSBequivalent=0
  Delay : Delay  DelayLength=1  InitialCondition=0
  Delay1 : Delay  DelayLength=1  InitialCondition=0
  From1 : From
  From3 : From
  Goto1 : Goto
  Integrator : Integrator
  MATLAB Function : MATLAB Function  TreatAsAtomicUnit=on
  MATLAB Function1 : MATLAB Function  TreatAsAtomicUnit=on
  MATLAB Function2 : MATLAB Function  TreatAsAtomicUnit=on
  Parallel RLC Branch : spsParallelRLCBranchLib/Parallel RLC Branch  LConnTagsString=a  RConnTagsString=__new0  BranchType=RC  Resistance=15.5e-3  Inductance=1e-3  SetiL0=off  InitialCurrent=0  Capacitance=1028.7  Setx0=off  InitialVoltage=0  Measurements=None
  Parallel RLC Branch1 : spsParallelRLCBranchLib/Parallel RLC Branch  LConnTagsString=a  RConnTagsString=__new0  BranchType=RC  Resistance=18.3e-3  Inductance=1e-3  SetiL0=off  InitialCurrent=0  Capacitance=5756.6  Setx0=off  InitialVoltage=0  Measurements=None
  Parallel RLC Branch2 : spsParallelRLCBranchLib/Parallel RLC Branch  LConnTagsString=a  RConnTagsString=__new0  BranchType=R  Resistance=1e9  Inductance=1e-3  SetiL0=off  InitialCurrent=0  Capacitance=5756.6  Setx0=off  InitialVoltage=0  Measurements=None
  Scope2 : Scope
  Scope3 : Scope
  Scope4 : Scope
  Variable Resistor : spsVariableResistorLib/Variable Resistor  Rabsmin=1e-3
      settings: LibrarySourceBlock=sps_lib/Passives/Variable Resistor
  Voltage Measurement1 : spsVoltageMeasurementLib/Voltage Measurement  PhasorSimulation=off  OutputType=Complex  PSBequivalent=0
  XY Graph : Record  FileSettingsInternal="{\"entries\":[{\"content\":{\"excelSettings\":{\"content\":{},\"type\":\"Streamout.ExcelSettings\"}},\"type\":\"Streamout.FileSettingStorage\",\"uuid\":\"33cd7e7e-cb3e-43fd-8af6-a1cd50dbb10c\"}],\"packageUris\":[\"http://schema.mathworks.com/mf0/streamout_blocks/R2020a\"],\"version\":\"1.0\"}"  Layout=[1 1]  SignalsInternal="{\"entries\":[{\"content\":{\"signals\":[{\"content\":{\"blockPath\":[\"untitled/Subsystem14/XY Graph\"],\"dimensions\":[1],\"domain\":\"untitled/Subsystem14/XY Graph\",\"lineColor\":\"#edb120\",\"port\":1,\"signalID\":758,\"signalName\":\"MATLAB Function2\"},\"type\":\"RecordBlkView.Signal\",\"uuid\":\"8d895311-2c35-4cbd-8deb-b3bbf5e6af65\"},{\"content\":{\"blockPath\":[\"untitled/Subsystem14/XY Graph\"],\"dimensions\":[1],\"domain\":\"untitled/Subsystem14/XY Graph\",\"lineColor\":\"#7e2f8e\",\"port\":2,\"signalID\":761,\"signalName\":\"Voltage Measurement1\"},\"type\":\"RecordBlkView.Signal\",\"uuid\":\"c8704904-ac01-4b23-b785-d814eb32b585\"}]},\"type\":\"RecordBlkView.InputSignals\",\"uuid\":\"24ffd32b-dee3-4fd5-8e55-47aa3769188f\"}],\"packageUris\":[\"http://schema.mathworks.com/mf0/streamout_blocks/R2020a\"],\"version\":\"1.0\"}"  VisualizationBindings="{\"xyplotplugin\":{\"info\":[{\"series\":[],\"subplotID\":1}]}}"  CompatibilityTag=XY
  powergui1 : spspowerguiLib/powergui  Priority=1  SimulationMode=Discrete  SampleTime=2e-7  frequency=60  Iterations=50  frequencyindice=0  Pbase=100e6  ErrMax=1e-4  UnitsV=kV  UnitsW=MW  buscounter=0  FunctionMessages=off  echomessages=off  EnableUseOfTLC=off  CurrentSourceSwitches=off  DisableSnubberDevices=off  DisableRonSwitches=off  DisableVfSwitches=off  DisplayEquations=off  AutomaticDiscreteSolvers=off  SolverType=Tustin/Backward Euler (TBE)  Interpol=off  ExternalGateDelay=off  methode=off  Ts=100  x0status=blocks  SPID=on  SwTol=0  HookPort=off  NonlinearTolerance=1e-4  nMaxIteration=100  ContinueOnMaxIteration=off  RestoreLinks=warning  ResistiveCurrentMeasurement=off  Frange=[0:2:500]  Ylog=off  Xlog=on  ShowGrid=off  save=off  variable=ZData  structure=0  ZoomFFT=off  StartTime=0.0  cycles=1  DisplayStyle=1  fundamental=60  FreqAxis=off  MaxFrequency=1000  frequencyindicesteady=1  RmsSteady=1  display=off
  + : PMIOPort  Side=Right
  - : PMIOPort  Port=2  Side=Left
  wires:
  Current Measurement/1 -> Goto1/1
  From3/1 -> Scope3/1
  Voltage Measurement1/1 -> XY Graph/2, Scope2/1
  MATLAB Function2/1(SOC) -> Delay/1, XY Graph/1, Scope4/1
  From1/1 -> Integrator/1
  MATLAB Function/1(y) -> Controlled Voltage Source/1
  MATLAB Function1/1(y) -> Variable Resistor/1
  Integrator/1 -> MATLAB Function2/1(u), MATLAB Function/1(u)
  Clock/1 -> MATLAB Function2/2(time), MATLAB Function/2(time)
  MATLAB Function/2(SOC) -> Delay1/1, MATLAB Function1/1(SOC)
  Delay/1 -> MATLAB Function2/3(SOC1)
  Delay1/1 -> MATLAB Function/3(SOC1)
  connections:
  Variable Resistor/RConn1 -- Parallel RLC Branch/LConn1
  Parallel RLC Branch1/RConn1 -- Parallel RLC Branch2/LConn1 -- +/RConn1 -- Voltage Measurement1/LConn1
  Voltage Measurement1/LConn2 -- Parallel RLC Branch2/RConn1 -- -/RConn1 -- Current Measurement/LConn1
  Controlled Voltage Source/RConn1 -- Variable Resistor/LConn1
  Current Measurement/RConn1 -- Controlled Voltage Source/LConn1
  Parallel RLC Branch/RConn1 -- Parallel RLC Branch1/LConn1

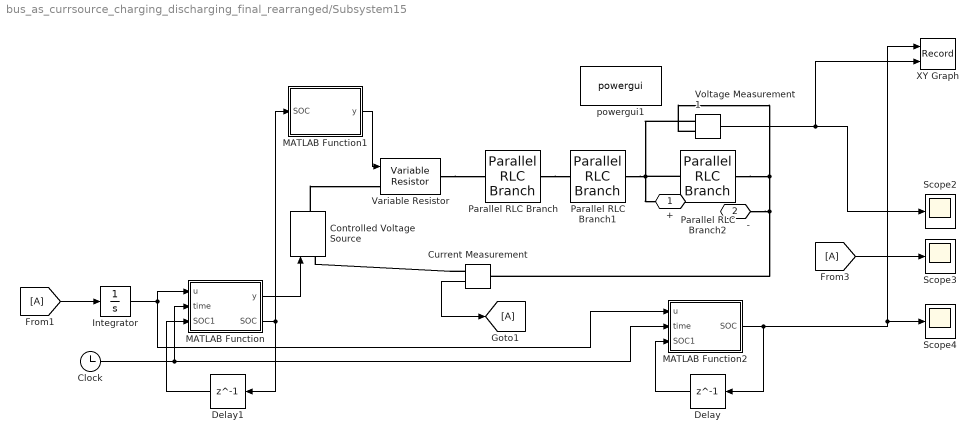
== system bus_as_currsource_charging_discharging_final_rearranged/Subsystem15 ==
  Clock : Clock
  Controlled Voltage Source : spsControlledVoltageSourceLib/Controlled Voltage Source  Initialize=on  Source_Type=DC  Amplitude=0  Phase=0  Frequency=0  Measurements=None
  Current Measurement : spsCurrentMeasurementLib/Current Measurement  PhasorSimulation=off  OutputType=Complex  PSBequivalent=0
  Delay : Delay  DelayLength=1  InitialCondition=0
  Delay1 : Delay  DelayLength=1  InitialCondition=0
  From1 : From
  From3 : From
  Goto1 : Goto
  Integrator : Integrator
  MATLAB Function : MATLAB Function  TreatAsAtomicUnit=on
  MATLAB Function1 : MATLAB Function  TreatAsAtomicUnit=on
  MATLAB Function2 : MATLAB Function  TreatAsAtomicUnit=on
  Parallel RLC Branch : spsParallelRLCBranchLib/Parallel RLC Branch  LConnTagsString=a  RConnTagsString=__new0  BranchType=RC  Resistance=15.5e-3  Inductance=1e-3  SetiL0=off  InitialCurrent=0  Capacitance=1028.7  Setx0=off  InitialVoltage=0  Measurements=None
  Parallel RLC Branch1 : spsParallelRLCBranchLib/Parallel RLC Branch  LConnTagsString=a  RConnTagsString=__new0  BranchType=RC  Resistance=18.3e-3  Inductance=1e-3  SetiL0=off  InitialCurrent=0  Capacitance=5756.6  Setx0=off  InitialVoltage=0  Measurements=None
  Parallel RLC Branch2 : spsParallelRLCBranchLib/Parallel RLC Branch  LConnTagsString=a  RConnTagsString=__new0  BranchType=R  Resistance=1e9  Inductance=1e-3  SetiL0=off  InitialCurrent=0  Capacitance=5756.6  Setx0=off  InitialVoltage=0  Measurements=None
  Scope2 : Scope
  Scope3 : Scope
  Scope4 : Scope
  Variable Resistor : spsVariableResistorLib/Variable Resistor  Rabsmin=1e-3
      settings: LibrarySourceBlock=sps_lib/Passives/Variable Resistor
  Voltage Measurement1 : spsVoltageMeasurementLib/Voltage Measurement  PhasorSimulation=off  OutputType=Complex  PSBequivalent=0
  XY Graph : Record  FileSettingsInternal="{\"entries\":[{\"content\":{\"excelSettings\":{\"content\":{},\"type\":\"Streamout.ExcelSettings\"}},\"type\":\"Streamout.FileSettingStorage\",\"uuid\":\"403cc223-e81b-4aa3-ab44-486a1f29fc47\"}],\"packageUris\":[\"http://schema.mathworks.com/mf0/streamout_blocks/R2020a\"],\"version\":\"1.0\"}"  Layout=[1 1]  SignalsInternal="{\"entries\":[{\"content\":{\"signals\":[{\"content\":{\"blockPath\":[\"untitled/Subsystem15/XY Graph\"],\"dimensions\":[1],\"domain\":\"untitled/Subsystem15/XY Graph\",\"lineColor\":\"#77ac30\",\"port\":1,\"signalID\":766,\"signalName\":\"MATLAB Function2\"},\"type\":\"RecordBlkView.Signal\",\"uuid\":\"c1a02276-32d7-41d4-a72a-c0476e60f96a\"},{\"content\":{\"blockPath\":[\"untitled/Subsystem15/XY Graph\"],\"dimensions\":[1],\"domain\":\"untitled/Subsystem15/XY Graph\",\"lineColor\":\"#4dbeee\",\"port\":2,\"signalID\":769,\"signalName\":\"Voltage Measurement1\"},\"type\":\"RecordBlkView.Signal\",\"uuid\":\"275a4661-1bcd-43c3-94eb-8eab3d22e323\"}]},\"type\":\"RecordBlkView.InputSignals\",\"uuid\":\"257ef280-70f4-4a70-9552-3d2113a1f719\"}],\"packageUris\":[\"http://schema.mathworks.com/mf0/streamout_blocks/R2020a\"],\"version\":\"1.0\"}"  VisualizationBindings="{\"xyplotplugin\":{\"info\":[{\"series\":[],\"subplotID\":1}]}}"  CompatibilityTag=XY
  powergui1 : spspowerguiLib/powergui  Priority=1  SimulationMode=Discrete  SampleTime=2e-7  frequency=60  Iterations=50  frequencyindice=0  Pbase=100e6  ErrMax=1e-4  UnitsV=kV  UnitsW=MW  buscounter=0  FunctionMessages=off  echomessages=off  EnableUseOfTLC=off  CurrentSourceSwitches=off  DisableSnubberDevices=off  DisableRonSwitches=off  DisableVfSwitches=off  DisplayEquations=off  AutomaticDiscreteSolvers=off  SolverType=Tustin/Backward Euler (TBE)  Interpol=off  ExternalGateDelay=off  methode=off  Ts=100  x0status=blocks  SPID=on  SwTol=0  HookPort=off  NonlinearTolerance=1e-4  nMaxIteration=100  ContinueOnMaxIteration=off  RestoreLinks=warning  ResistiveCurrentMeasurement=off  Frange=[0:2:500]  Ylog=off  Xlog=on  ShowGrid=off  save=off  variable=ZData  structure=0  ZoomFFT=off  StartTime=0.0  cycles=1  DisplayStyle=1  fundamental=60  FreqAxis=off  MaxFrequency=1000  frequencyindicesteady=1  RmsSteady=1  display=off
  + : PMIOPort  Side=Right
  - : PMIOPort  Port=2  Side=Left
  wires:
  Current Measurement/1 -> Goto1/1
  From3/1 -> Scope3/1
  Voltage Measurement1/1 -> XY Graph/2, Scope2/1
  MATLAB Function2/1(SOC) -> Delay/1, XY Graph/1, Scope4/1
  From1/1 -> Integrator/1
  MATLAB Function/1(y) -> Controlled Voltage Source/1
  MATLAB Function1/1(y) -> Variable Resistor/1
  Integrator/1 -> MATLAB Function2/1(u), MATLAB Function/1(u)
  Clock/1 -> MATLAB Function2/2(time), MATLAB Function/2(time)
  MATLAB Function/2(SOC) -> Delay1/1, MATLAB Function1/1(SOC)
  Delay/1 -> MATLAB Function2/3(SOC1)
  Delay1/1 -> MATLAB Function/3(SOC1)
  connections:
  Variable Resistor/RConn1 -- Parallel RLC Branch/LConn1
  Parallel RLC Branch1/RConn1 -- Parallel RLC Branch2/LConn1 -- +/RConn1 -- Voltage Measurement1/LConn1
  Voltage Measurement1/LConn2 -- Parallel RLC Branch2/RConn1 -- -/RConn1 -- Current Measurement/LConn1
  Controlled Voltage Source/RConn1 -- Variable Resistor/LConn1
  Current Measurement/RConn1 -- Controlled Voltage Source/LConn1
  Parallel RLC Branch/RConn1 -- Parallel RLC Branch1/LConn1

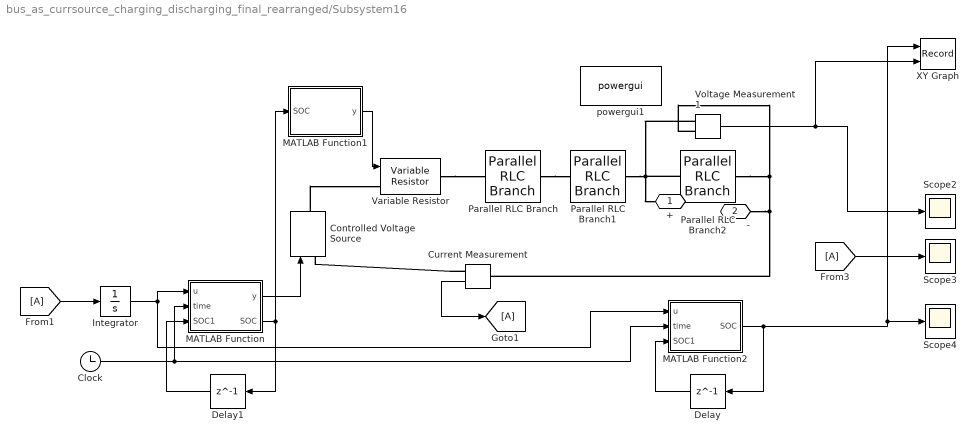
== system bus_as_currsource_charging_discharging_final_rearranged/Subsystem16 ==
  Clock : Clock
  Controlled Voltage Source : spsControlledVoltageSourceLib/Controlled Voltage Source  Initialize=on  Source_Type=DC  Amplitude=0  Phase=0  Frequency=0  Measurements=None
  Current Measurement : spsCurrentMeasurementLib/Current Measurement  PhasorSimulation=off  OutputType=Complex  PSBequivalent=0
  Delay : Delay  DelayLength=1  InitialCondition=0
  Delay1 : Delay  DelayLength=1  InitialCondition=0
  From1 : From
  From3 : From
  Goto1 : Goto
  Integrator : Integrator
  MATLAB Function : MATLAB Function  TreatAsAtomicUnit=on
  MATLAB Function1 : MATLAB Function  TreatAsAtomicUnit=on
  MATLAB Function2 : MATLAB Function  TreatAsAtomicUnit=on
  Parallel RLC Branch : spsParallelRLCBranchLib/Parallel RLC Branch  LConnTagsString=a  RConnTagsString=__new0  BranchType=RC  Resistance=15.5e-3  Inductance=1e-3  SetiL0=off  InitialCurrent=0  Capacitance=1028.7  Setx0=off  InitialVoltage=0  Measurements=None
  Parallel RLC Branch1 : spsParallelRLCBranchLib/Parallel RLC Branch  LConnTagsString=a  RConnTagsString=__new0  BranchType=RC  Resistance=18.3e-3  Inductance=1e-3  SetiL0=off  InitialCurrent=0  Capacitance=5756.6  Setx0=off  InitialVoltage=0  Measurements=None
  Parallel RLC Branch2 : spsParallelRLCBranchLib/Parallel RLC Branch  LConnTagsString=a  RConnTagsString=__new0  BranchType=R  Resistance=1e9  Inductance=1e-3  SetiL0=off  InitialCurrent=0  Capacitance=5756.6  Setx0=off  InitialVoltage=0  Measurements=None
  Scope2 : Scope
  Scope3 : Scope
  Scope4 : Scope
  Variable Resistor : spsVariableResistorLib/Variable Resistor  Rabsmin=1e-3
      settings: LibrarySourceBlock=sps_lib/Passives/Variable Resistor
  Voltage Measurement1 : spsVoltageMeasurementLib/Voltage Measurement  PhasorSimulation=off  OutputType=Complex  PSBequivalent=0
  XY Graph : Record  FileSettingsInternal="{\"entries\":[{\"content\":{\"excelSettings\":{\"content\":{},\"type\":\"Streamout.ExcelSettings\"}},\"type\":\"Streamout.FileSettingStorage\",\"uuid\":\"635a8de4-9d68-4305-8374-c64c95cd4a88\"}],\"packageUris\":[\"http://schema.mathworks.com/mf0/streamout_blocks/R2020a\"],\"version\":\"1.0\"}"  Layout=[1 1]  SignalsInternal="{\"entries\":[{\"content\":{\"signals\":[{\"content\":{\"blockPath\":[\"untitled/Subsystem16/XY Graph\"],\"dimensions\":[1],\"domain\":\"untitled/Subsystem16/XY Graph\",\"lineColor\":\"#a2142f\",\"port\":1,\"signalID\":774,\"signalName\":\"MATLAB Function2\"},\"type\":\"RecordBlkView.Signal\",\"uuid\":\"4a7bc012-1bee-4532-adb5-a858f4fb98a9\"},{\"content\":{\"blockPath\":[\"untitled/Subsystem16/XY Graph\"],\"dimensions\":[1],\"domain\":\"untitled/Subsystem16/XY Graph\",\"lineColor\":\"#139fff\",\"port\":2,\"signalID\":777,\"signalName\":\"Voltage Measurement1\"},\"type\":\"RecordBlkView.Signal\",\"uuid\":\"7f67f342-12e1-4167-85bc-002c2461bfa9\"}]},\"type\":\"RecordBlkView.InputSignals\",\"uuid\":\"2abac92f-8a54-481c-8c63-d11d4257a30b\"}],\"packageUris\":[\"http://schema.mathworks.com/mf0/streamout_blocks/R2020a\"],\"version\":\"1.0\"}"  VisualizationBindings="{\"xyplotplugin\":{\"info\":[{\"series\":[],\"subplotID\":1}]}}"  CompatibilityTag=XY
  powergui1 : spspowerguiLib/powergui  Priority=1  SimulationMode=Discrete  SampleTime=2e-7  frequency=60  Iterations=50  frequencyindice=0  Pbase=100e6  ErrMax=1e-4  UnitsV=kV  UnitsW=MW  buscounter=0  FunctionMessages=off  echomessages=off  EnableUseOfTLC=off  CurrentSourceSwitches=off  DisableSnubberDevices=off  DisableRonSwitches=off  DisableVfSwitches=off  DisplayEquations=off  AutomaticDiscreteSolvers=off  SolverType=Tustin/Backward Euler (TBE)  Interpol=off  ExternalGateDelay=off  methode=off  Ts=100  x0status=blocks  SPID=on  SwTol=0  HookPort=off  NonlinearTolerance=1e-4  nMaxIteration=100  ContinueOnMaxIteration=off  RestoreLinks=warning  ResistiveCurrentMeasurement=off  Frange=[0:2:500]  Ylog=off  Xlog=on  ShowGrid=off  save=off  variable=ZData  structure=0  ZoomFFT=off  StartTime=0.0  cycles=1  DisplayStyle=1  fundamental=60  FreqAxis=off  MaxFrequency=1000  frequencyindicesteady=1  RmsSteady=1  display=off
  + : PMIOPort  Side=Right
  - : PMIOPort  Port=2  Side=Left
  wires:
  Current Measurement/1 -> Goto1/1
  From3/1 -> Scope3/1
  Voltage Measurement1/1 -> XY Graph/2, Scope2/1
  MATLAB Function2/1(SOC) -> Delay/1, XY Graph/1, Scope4/1
  From1/1 -> Integrator/1
  MATLAB Function/1(y) -> Controlled Voltage Source/1
  MATLAB Function1/1(y) -> Variable Resistor/1
  Integrator/1 -> MATLAB Function2/1(u), MATLAB Function/1(u)
  Clock/1 -> MATLAB Function2/2(time), MATLAB Function/2(time)
  MATLAB Function/2(SOC) -> Delay1/1, MATLAB Function1/1(SOC)
  Delay/1 -> MATLAB Function2/3(SOC1)
  Delay1/1 -> MATLAB Function/3(SOC1)
  connections:
  Variable Resistor/RConn1 -- Parallel RLC Branch/LConn1
  Parallel RLC Branch1/RConn1 -- Parallel RLC Branch2/LConn1 -- +/RConn1 -- Voltage Measurement1/LConn1
  Voltage Measurement1/LConn2 -- Parallel RLC Branch2/RConn1 -- -/RConn1 -- Current Measurement/LConn1
  Controlled Voltage Source/RConn1 -- Variable Resistor/LConn1
  Current Measurement/RConn1 -- Controlled Voltage Source/LConn1
  Parallel RLC Branch/RConn1 -- Parallel RLC Branch1/LConn1
